simulink library "ALD1105"  (R2016a)
settings: Solver=ode45  StartTime=0.0  StopTime=10.0  RelTol=1e-3
libraries: fl_lib x14, elec_lib x8
settings Model: Creator=Peter  LastModifiedBy=Peter
settings DataIOCC: LimitDataPoints=on
settings DebuggingCC: AllowSymbolicDim=off

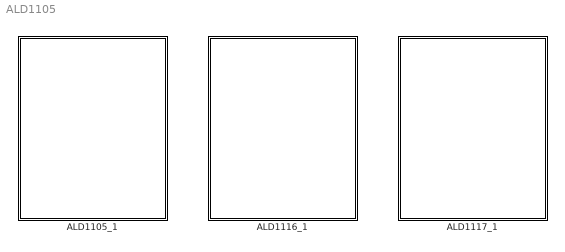
== system ALD1105 ==
  ALD1105_1 : Subsystem
      mask Display: image('ALD1105.png');
  ALD1116_1 : Subsystem
      mask Display: image('ALD1116.png');
  ALD1117_1 : Subsystem
      mask Display: image('ALD1117.png');

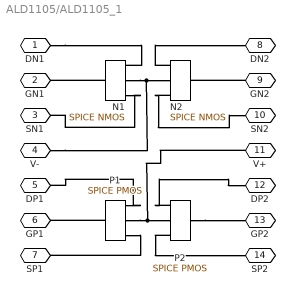
== system ALD1105/ALD1105_1 ==
  N1 : elec_lib/Additional Components/SPICE-Compatible Components/Semiconductor Devices/SPICE NMOS  AREA=1  SCALE=1  LENGTH=7.8e-6 m  WIDTH=0.138e-3 m  AD=0.161e-8 m^2  AS=0.603e-8 m^2  PD=0 m  PS=0.478e-3 m  NRD=0.3  NRS=1  LEVEL=1  VTO=0.750 V  KP=NaN A/V^2  GAMMA=1.03 V^0.50000  PHI=0.70 V  LAMBDA=0.018 1/V  RD=NaN Ohm  RS=NaN Ohm  C_param=1  CBD=1e-18 F  CBS=1e-18 F  IS=1.206e-13 A  ND=1  PB=0.9 V  CGSO=0.94e-9 F/m  CGDO=0.59e-9 F/m  CGBO=0.138e-9 F/m  RSH=10 Ohm  CJ=0.39e-3 F/m^2  MJ=0.5  CJSW=264e-12 F/m  MJSW=0.18  JS=20e-6 A/m^2  TOX=0.055e-6 m  LD=1.6e-6 m  U0=650 cm^2/s/V  FC=0.5  NSUB=1e16 1/cm^3  TPG=1  NSS=0.7e11 1/cm^2  UEXP=0  UCRIT=1e+4 V/cm  NEFF=1  DELTA=0  VMAX=1.6e5 m/s  XJ=2.0e-6 m  NFS=1.17e11 1/cm^2  ETA=0  THETA=0 1/V  KAPPA=0.2  T_param=1  TOFFSET=0 K  TFIXED=300.15 K  TMEAS=300.15 K  IC_given=1  ICVDS=0 V  ICVGS=0 V  ICVBS=0 V  MTYPE=1
  N2 : elec_lib/Additional Components/SPICE-Compatible Components/Semiconductor Devices/SPICE NMOS  AREA=1  SCALE=1  LENGTH=7.8e-6 m  WIDTH=0.138e-3 m  AD=0.161e-8 m^2  AS=0.603e-8 m^2  PD=0 m  PS=0.478e-3 m  NRD=0.3  NRS=1  LEVEL=1  VTO=0.750 V  KP=NaN A/V^2  GAMMA=1.03 V^0.50000  PHI=0.70 V  LAMBDA=0.018 1/V  RD=NaN Ohm  RS=NaN Ohm  C_param=1  CBD=1e-18 F  CBS=1e-18 F  IS=1.206e-13 A  ND=1  PB=0.9 V  CGSO=0.94e-9 F/m  CGDO=0.59e-9 F/m  CGBO=0.138e-9 F/m  RSH=10 Ohm  CJ=0.39e-3 F/m^2  MJ=0.5  CJSW=264e-12 F/m  MJSW=0.18  JS=20e-6 A/m^2  TOX=0.055e-6 m  LD=1.6e-6 m  U0=650 cm^2/s/V  FC=0.5  NSUB=1e16 1/cm^3  TPG=1  NSS=0.7e11 1/cm^2  UEXP=0  UCRIT=1e+4 V/cm  NEFF=1  DELTA=0  VMAX=1.6e5 m/s  XJ=2.0e-6 m  NFS=1.17e11 1/cm^2  ETA=0  THETA=0 1/V  KAPPA=0.2  T_param=1  TOFFSET=0 K  TFIXED=300.15 K  TMEAS=300.15 K  IC_given=1  ICVDS=0 V  ICVGS=0 V  ICVBS=0 V  MTYPE=1
  P1 : elec_lib/Additional Components/SPICE-Compatible Components/Semiconductor Devices/SPICE PMOS  AREA=1  SCALE=1  LENGTH=7.8e-6 m  WIDTH=0.138e-3 m  AD=0.161e-8 m^2  AS=0.603e-8 m^2  PD=0 m  PS=0.478e-3 m  NRD=0.3  NRS=1  LEVEL=1  VTO=-0.74 V  KP=NaN A/V^2  GAMMA=0.58 V^0.50000  PHI=0.70 V  LAMBDA=.026 1/V  RD=NaN Ohm  RS=NaN Ohm  C_param=1  CBD=1e-18 F  CBS=1e-18 F  IS=1.206e-13 A  ND=1  PB=0.90 V  CGSO=0.31e-9 F/m  CGDO=0.39e-9 F/m  CGBO=0.138e-9 F/m  RSH=90 Ohm  CJ=0.18e-3 F/m^2  MJ=0.57  CJSW=322e-12 F/m  MJSW=0.33  JS=20e-6 A/m^2  TOX=0.055e-6 m  LD=0.96e-6 m  U0=260 cm^2/s/V  FC=0.5  NSUB=1e16 1/cm^3  TPG=-1  NSS=1e11 1/cm^2  UEXP=0  UCRIT=1e+4 V/cm  NEFF=1  DELTA=0  VMAX=3.0e5 m/s  XJ=1.2e-6 m  NFS=1.06e11 1/cm^2  ETA=0  THETA=0 1/V  KAPPA=0.2  T_param=1  TOFFSET=0 K  TFIXED=300.15 K  TMEAS=300.15 K  IC_given=1  ICVDS=0 V  ICVGS=0 V  ICVBS=0 V  MTYPE=-1
  P2 : elec_lib/Additional Components/SPICE-Compatible Components/Semiconductor Devices/SPICE PMOS  AREA=1  SCALE=1  LENGTH=7.8e-6 m  WIDTH=0.138e-3 m  AD=0.161e-8 m^2  AS=0.603e-8 m^2  PD=0 m  PS=0.478e-3 m  NRD=0.3  NRS=1  LEVEL=1  VTO=-0.74 V  KP=NaN A/V^2  GAMMA=0.58 V^0.50000  PHI=0.70 V  LAMBDA=.026 1/V  RD=NaN Ohm  RS=NaN Ohm  C_param=1  CBD=1e-18 F  CBS=1e-18 F  IS=1.206e-13 A  ND=1  PB=0.90 V  CGSO=0.31e-9 F/m  CGDO=0.39e-9 F/m  CGBO=0.138e-9 F/m  RSH=90 Ohm  CJ=0.18e-3 F/m^2  MJ=0.57  CJSW=322e-12 F/m  MJSW=0.33  JS=20e-6 A/m^2  TOX=0.055e-6 m  LD=0.96e-6 m  U0=260 cm^2/s/V  FC=0.5  NSUB=1e16 1/cm^3  TPG=-1  NSS=1e11 1/cm^2  UEXP=0  UCRIT=1e+4 V/cm  NEFF=1  DELTA=0  VMAX=3.0e5 m/s  XJ=1.2e-6 m  NFS=1.06e11 1/cm^2  ETA=0  THETA=0 1/V  KAPPA=0.2  T_param=1  TOFFSET=0 K  TFIXED=300.15 K  TMEAS=300.15 K  IC_given=1  ICVDS=0 V  ICVGS=0 V  ICVBS=0 V  MTYPE=-1
  DN1 : PMIOPort  Port=1  Side=Left
  GN1 : PMIOPort  Port=2  Side=Left
  SN1 : PMIOPort  Port=3  Side=Left
  V- : PMIOPort  Port=4  Side=Left
  DP1 : PMIOPort  Port=5  Side=Left
  GP1 : PMIOPort  Port=6  Side=Left
  SP1 : PMIOPort  Port=7  Side=Left
  DN2 : PMIOPort  Port=8  Side=Right
  GN2 : PMIOPort  Port=9  Side=Right
  SN2 : PMIOPort  Port=10  Side=Right
  V+ : PMIOPort  Port=11  Side=Right
  DP2 : PMIOPort  Port=12  Side=Right
  GP2 : PMIOPort  Port=13  Side=Right
  SP2 : PMIOPort  Port=14  Side=Right
  connections:
  N1/RConn2 -- N2/RConn2 -- V-/RConn1
  N1/LConn1 -- GN1/RConn1
  GN2/RConn1 -- N2/LConn1
  P1/LConn1 -- GP1/RConn1
  P2/LConn1 -- GP2/RConn1
  P2/RConn1 -- SP2/RConn1
  P1/RConn1 -- SP1/RConn1
  N1/RConn1 -- SN1/RConn1
  N2/RConn1 -- SN2/RConn1
  P1/RConn2 -- V+/RConn1 -- P2/RConn2
  P2/RConn3 -- DP2/RConn1
  P1/RConn3 -- DP1/RConn1
  DN1/RConn1 -- N1/RConn3
  N2/RConn3 -- DN2/RConn1

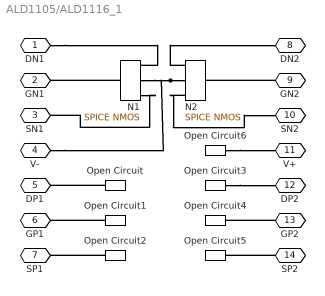
== system ALD1105/ALD1116_1 ==
  N1 : elec_lib/Additional Components/SPICE-Compatible Components/Semiconductor Devices/SPICE NMOS  AREA=1  SCALE=1  LENGTH=7.8e-6 m  WIDTH=0.138e-3 m  AD=0.161e-8 m^2  AS=0.603e-8 m^2  PD=0 m  PS=0.478e-3 m  NRD=0.3  NRS=1  LEVEL=1  VTO=0.750 V  KP=NaN A/V^2  GAMMA=1.03 V^0.50000  PHI=0.70 V  LAMBDA=0.018 1/V  RD=NaN Ohm  RS=NaN Ohm  C_param=1  CBD=1e-18 F  CBS=1e-18 F  IS=1.206e-13 A  ND=1  PB=0.9 V  CGSO=0.94e-9 F/m  CGDO=0.59e-9 F/m  CGBO=0.138e-9 F/m  RSH=10 Ohm  CJ=0.39e-3 F/m^2  MJ=0.5  CJSW=264e-12 F/m  MJSW=0.18  JS=20e-6 A/m^2  TOX=0.055e-6 m  LD=1.6e-6 m  U0=650 cm^2/s/V  FC=0.5  NSUB=1e16 1/cm^3  TPG=1  NSS=0.7e11 1/cm^2  UEXP=0  UCRIT=1e+4 V/cm  NEFF=1  DELTA=0  VMAX=1.6e5 m/s  XJ=2.0e-6 m  NFS=1.17e11 1/cm^2  ETA=0  THETA=0 1/V  KAPPA=0.2  T_param=1  TOFFSET=0 K  TFIXED=300.15 K  TMEAS=300.15 K  IC_given=1  ICVDS=0 V  ICVGS=0 V  ICVBS=0 V  MTYPE=1
  N2 : elec_lib/Additional Components/SPICE-Compatible Components/Semiconductor Devices/SPICE NMOS  AREA=1  SCALE=1  LENGTH=7.8e-6 m  WIDTH=0.138e-3 m  AD=0.161e-8 m^2  AS=0.603e-8 m^2  PD=0 m  PS=0.478e-3 m  NRD=0.3  NRS=1  LEVEL=1  VTO=0.750 V  KP=NaN A/V^2  GAMMA=1.03 V^0.50000  PHI=0.70 V  LAMBDA=0.018 1/V  RD=NaN Ohm  RS=NaN Ohm  C_param=1  CBD=1e-18 F  CBS=1e-18 F  IS=1.206e-13 A  ND=1  PB=0.9 V  CGSO=0.94e-9 F/m  CGDO=0.59e-9 F/m  CGBO=0.138e-9 F/m  RSH=10 Ohm  CJ=0.39e-3 F/m^2  MJ=0.5  CJSW=264e-12 F/m  MJSW=0.18  JS=20e-6 A/m^2  TOX=0.055e-6 m  LD=1.6e-6 m  U0=650 cm^2/s/V  FC=0.5  NSUB=1e16 1/cm^3  TPG=1  NSS=0.7e11 1/cm^2  UEXP=0  UCRIT=1e+4 V/cm  NEFF=1  DELTA=0  VMAX=1.6e5 m/s  XJ=2.0e-6 m  NFS=1.17e11 1/cm^2  ETA=0  THETA=0 1/V  KAPPA=0.2  T_param=1  TOFFSET=0 K  TFIXED=300.15 K  TMEAS=300.15 K  IC_given=1  ICVDS=0 V  ICVGS=0 V  ICVBS=0 V  MTYPE=1
  Open Circuit{,1..6} (7 alike) : fl_lib/Electrical/Electrical Elements/Open Circuit  v_specify=off  v_priority=None  v=0 V
  DN1 : PMIOPort  Port=1  Side=Left
  GN1 : PMIOPort  Port=2  Side=Left
  SN1 : PMIOPort  Port=3  Side=Left
  V- : PMIOPort  Port=4  Side=Left
  DP1 : PMIOPort  Port=5  Side=Left
  GP1 : PMIOPort  Port=6  Side=Left
  SP1 : PMIOPort  Port=7  Side=Left
  DN2 : PMIOPort  Port=8  Side=Right
  GN2 : PMIOPort  Port=9  Side=Right
  SN2 : PMIOPort  Port=10  Side=Right
  V+ : PMIOPort  Port=11  Side=Right
  DP2 : PMIOPort  Port=12  Side=Right
  GP2 : PMIOPort  Port=13  Side=Right
  SP2 : PMIOPort  Port=14  Side=Right
  connections:
  Open Circuit2/LConn1 -- SP1/RConn1
  GP2/RConn1 -- Open Circuit4/LConn1
  Open Circuit3/LConn1 -- DP2/RConn1
  Open Circuit/LConn1 -- DP1/RConn1
  SP2/RConn1 -- Open Circuit5/LConn1
  N1/RConn1 -- SN1/RConn1
  N2/RConn3 -- DN2/RConn1
  N2/RConn2 -- V-/RConn1 -- N1/RConn2
  N1/LConn1 -- GN1/RConn1
  GN2/RConn1 -- N2/LConn1
  N2/RConn1 -- SN2/RConn1
  DN1/RConn1 -- N1/RConn3
  Open Circuit1/LConn1 -- GP1/RConn1
  Open Circuit6/LConn1 -- V+/RConn1

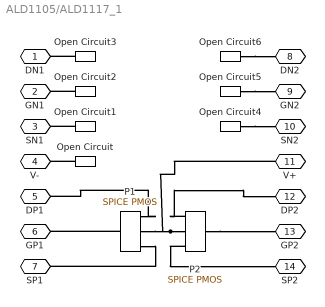
== system ALD1105/ALD1117_1 ==
  Open Circuit{,1..6} (7 alike) : fl_lib/Electrical/Electrical Elements/Open Circuit  v_specify=off  v_priority=None  v=0 V
  P1 : elec_lib/Additional Components/SPICE-Compatible Components/Semiconductor Devices/SPICE PMOS  AREA=1  SCALE=1  LENGTH=7.8e-6 m  WIDTH=0.138e-3 m  AD=0.161e-8 m^2  AS=0.603e-8 m^2  PD=0 m  PS=0.478e-3 m  NRD=0.3  NRS=1  LEVEL=1  VTO=-0.74 V  KP=NaN A/V^2  GAMMA=0.58 V^0.50000  PHI=0.70 V  LAMBDA=.026 1/V  RD=NaN Ohm  RS=NaN Ohm  C_param=2  CBD=1e-18 F  CBS=1e-18 F  IS=1.206e-13 A  ND=1  PB=0.90 V  CGSO=0.31e-9 F/m  CGDO=0.39e-9 F/m  CGBO=0.138e-9 F/m  RSH=90 Ohm  CJ=0.18e-3 F/m^2  MJ=0.57  CJSW=322e-12 F/m  MJSW=0.33  JS=20e-6 A/m^2  TOX=0.055e-6 m  LD=0.96e-6 m  U0=260 cm^2/s/V  FC=0.5  NSUB=1e16 1/cm^3  TPG=-1  NSS=1e11 1/cm^2  UEXP=0  UCRIT=1e+4 V/cm  NEFF=1  DELTA=0  VMAX=3.0e5 m/s  XJ=1.2e-6 m  NFS=1.06e11 1/cm^2  ETA=0  THETA=0 1/V  KAPPA=0.2  T_param=1  TOFFSET=0 K  TFIXED=300.15 K  TMEAS=300.15 K  IC_given=1  ICVDS=0 V  ICVGS=0 V  ICVBS=0 V  MTYPE=-1
  P2 : elec_lib/Additional Components/SPICE-Compatible Components/Semiconductor Devices/SPICE PMOS  AREA=1  SCALE=1  LENGTH=7.8e-6 m  WIDTH=0.138e-3 m  AD=0.161e-8 m^2  AS=0.603e-8 m^2  PD=0 m  PS=0.478e-3 m  NRD=0.3  NRS=1  LEVEL=1  VTO=-0.74 V  KP=NaN A/V^2  GAMMA=0.58 V^0.50000  PHI=0.70 V  LAMBDA=.026 1/V  RD=NaN Ohm  RS=NaN Ohm  C_param=2  CBD=1e-18 F  CBS=1e-18 F  IS=1.206e-13 A  ND=1  PB=0.90 V  CGSO=0.31e-9 F/m  CGDO=0.39e-9 F/m  CGBO=0.138e-9 F/m  RSH=90 Ohm  CJ=0.18e-3 F/m^2  MJ=0.57  CJSW=322e-12 F/m  MJSW=0.33  JS=20e-6 A/m^2  TOX=0.055e-6 m  LD=0.96e-6 m  U0=260 cm^2/s/V  FC=0.5  NSUB=1e16 1/cm^3  TPG=-1  NSS=1e11 1/cm^2  UEXP=0  UCRIT=1e+4 V/cm  NEFF=1  DELTA=0  VMAX=3.0e5 m/s  XJ=1.2e-6 m  NFS=1.06e11 1/cm^2  ETA=0  THETA=0 1/V  KAPPA=0.2  T_param=1  TOFFSET=0 K  TFIXED=300.15 K  TMEAS=300.15 K  IC_given=1  ICVDS=0 V  ICVGS=0 V  ICVBS=0 V  MTYPE=-1
  DN1 : PMIOPort  Port=1  Side=Left
  GN1 : PMIOPort  Port=2  Side=Left
  SN1 : PMIOPort  Port=3  Side=Left
  V- : PMIOPort  Port=4  Side=Left
  DP1 : PMIOPort  Port=5  Side=Left
  GP1 : PMIOPort  Port=6  Side=Left
  SP1 : PMIOPort  Port=7  Side=Left
  DN2 : PMIOPort  Port=8  Side=Right
  GN2 : PMIOPort  Port=9  Side=Right
  SN2 : PMIOPort  Port=10  Side=Right
  V+ : PMIOPort  Port=11  Side=Right
  DP2 : PMIOPort  Port=12  Side=Right
  GP2 : PMIOPort  Port=13  Side=Right
  SP2 : PMIOPort  Port=14  Side=Right
  connections:
  P2/RConn1 -- SP2/RConn1
  P2/RConn2 -- V+/RConn1 -- P1/RConn2
  P2/LConn1 -- GP2/RConn1
  P1/RConn1 -- SP1/RConn1
  P1/LConn1 -- GP1/RConn1
  P2/RConn3 -- DP2/RConn1
  P1/RConn3 -- DP1/RConn1
  Open Circuit/LConn1 -- V-/RConn1
  Open Circuit1/LConn1 -- SN1/RConn1
  Open Circuit2/LConn1 -- GN1/RConn1
  Open Circuit3/LConn1 -- DN1/RConn1
  Open Circuit6/LConn1 -- DN2/RConn1
  Open Circuit5/LConn1 -- GN2/RConn1
  Open Circuit4/LConn1 -- SN2/RConn1
